simulink model "mymodel"  (R2023b)
settings: Solver=VariableStepAuto  StartTime=0.0  StopTime=10.0  RelTol=1e-3
undefined symbols (not defined in the file or in its folder): SS_lat_lo8
libraries: simulink_extras x2
settings Model: Creator=antonhendrickx  LastModifiedBy=antonhendrickx

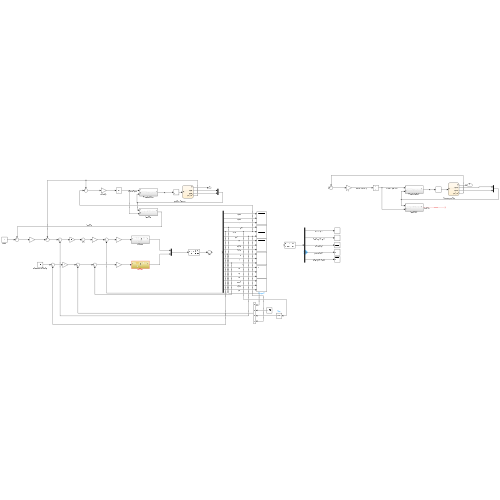
[thumbnail: Simulink's stored preview of the top-level diagram]
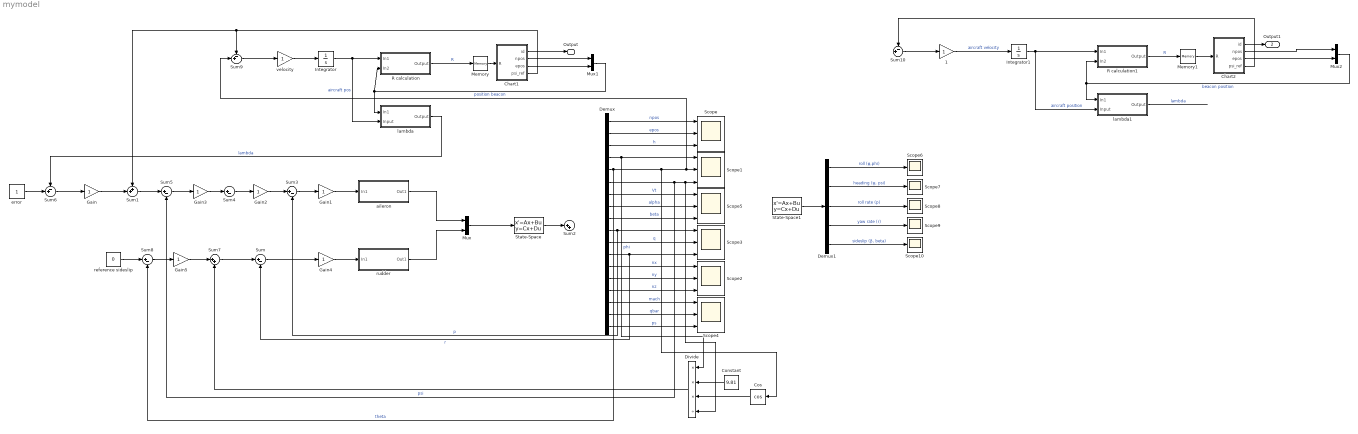
== system mymodel ==
  1 : Gain
  Chart1 : Stateflow chart  TreatAsAtomicUnit=on
  Chart2 : Stateflow chart  TreatAsAtomicUnit=on
  Constant : Constant  Value=9.81
  Cos : Trigonometry  Operator=cos
  Demux : Demux  Outputs=18
  Demux1 : Demux  Outputs=5
  Divide : Product  Inputs=***/
  Gain{,1..5} (6 alike) : Gain
  Integrator : Integrator
  Integrator1 : Integrator
  Memory : Memory
  Memory1 : Memory
  Mux : Mux  Inputs=2
  Mux1 : Mux  Inputs=2
  Mux2 : Mux  Inputs=2
  R calculation : Subsystem
  R calculation1 : Subsystem
  Scope{,1..5} (6 alike) : Scope  NumInputPorts=3
  Scope{6..10} (5 alike) : Scope
  State-Space : StateSpace  A=SS_lat_lo8.A  B=SS_lat_lo8.B  C=SS_lat_lo8.C  D=SS_lat_lo8.D  InitialCondition=0
  State-Space1 : StateSpace  InitialCondition=0
  Sum{,3..5,8} (5 alike) : Sum  Inputs=|+-
  Sum1 : Sum  Inputs=++|
  Sum10 : Sum  Inputs=-+|
  Sum2 : Sum  Inputs=|++
  Sum6 : Sum  Inputs=-+|
  Sum7 : Sum  Inputs=|++
  Sum9 : Sum  Inputs=-+|
  aileron : Subsystem
  error : Constant
  lambda : Subsystem
  lambda1 : Subsystem
  reference sideslip : Constant  Value=0
  rudder : Subsystem
  velocity : Gain
  Output : Outport
  Output1 : Outport  Port=2
  wires:
  Gain/1 -> Sum1/2
  Mux/1 -> State-Space/1
  aileron/1(Out1) -> Mux/1
  rudder/1(Out1) -> Mux/2
  Gain1/1 -> aileron/1(In1)
  Sum3/1 -> Gain1/1
  Gain2/1 -> Sum3/1
  Sum4/1 -> Gain2/1
  Gain3/1 -> Sum4/1
  Sum5/1 -> Gain3/1
  error/1 -> Sum6/2
  Sum6/1 -> Gain/1
  Sum1/1 -> Sum5/1
  Gain4/1 -> rudder/1(In1)
  Sum/1 -> Gain4/1
  Sum7/1 -> Sum/1
  Gain5/1 -> Sum7/1
  reference sideslip/1 -> Sum8/1
  Sum8/1 -> Gain5/1
  Demux/1 -> Scope/1  "npos"
  Demux/2 -> Scope/2  "epos"
  Demux/3 -> Scope/3  "h"
  Demux/4 -> Divide/1, Scope1/1  "phi"
  Demux/5 -> Sum8/2, Cos/1, Scope1/2, Sum9/2  "theta"
  Demux/6 -> Divide/4, Scope1/3, Sum5/2  "psi"
  Demux/7 -> Scope5/1  "Vt"
  Demux/8 -> Scope5/2  "alpha"
  Demux/9 -> Scope5/3  "beta"
  Demux/10 -> Sum3/2, Scope3/1  "p"
  Demux/11 -> Scope3/2  "q"
  Demux/12 -> Scope3/3, Sum/2  "r"
  Demux/13 -> Scope2/1  "nx"
  Demux/14 -> Scope2/2  "ny"
  Demux/15 -> Scope2/3  "nz"
  Demux/16 -> Scope4/1  "mach"
  Demux/17 -> Scope4/2  "qbar"
  Demux/18 -> Scope4/3  "ps"
  Chart1/1(id) -> Output/1
  Chart1/2(npos) -> Mux1/1
  Memory/1 -> Chart1/1(R)
  Chart1/3(epos) -> Mux1/2
  Sum9/1 -> velocity/1
  velocity/1 -> Integrator/1
  Integrator/1 -> lambda/2(Input), R calculation/1(In1)  "aircraft pos"
  Chart1/4(psi_ref) -> Sum9/1, Sum1/1
  Mux1/1 -> lambda/1(In1), R calculation/2(In2)  "position beacon"
  R calculation/1(Output) -> Memory/1  "R"
  lambda/1(Output) -> Sum6/1  "lambda"
  Divide/1 -> Sum7/2
  Constant/1 -> Divide/2
  Cos/1 -> Divide/3
  State-Space/1 -> Sum2/1
  Demux1/1 -> Scope6/1  "roll (φ,phi)"
  Demux1/2 -> Scope7/1  "heading (ψ, psi)"
  Demux1/3 -> Scope8/1  "roll rate (p)"
  Demux1/4 -> Scope9/1  "yaw rate (r)"
  Demux1/5 -> Scope10/1  "sideslip (β, beta)"
  State-Space1/1 -> Demux1/1
  Integrator1/1 -> lambda1/2(Input), R calculation1/1(In1)  "aircraft position"
  1/1 -> Integrator1/1  "aircraft velocity"
  Memory1/1 -> Chart2/1(R)
  R calculation1/1(Output) -> Memory1/1  "R"
  Chart2/1(id) -> Output1/1
  Chart2/2(npos) -> Mux2/1
  Chart2/3(epos) -> Mux2/2
  Chart2/4(psi_ref) -> Sum10/1
  Sum10/1 -> 1/1
  Mux2/1 -> lambda1/1(In1), R calculation1/2(In2)  "beacon position"
  lambda1/1(Output) -> ?  "lambda"

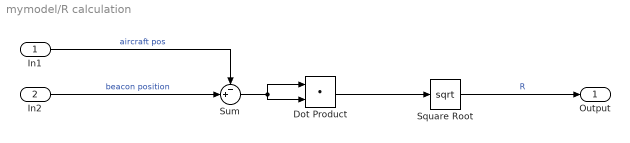
== system mymodel/R calculation ==
  In1 : Inport
  In2 : Inport  Port=2
  Dot Product : DotProduct  OutDataTypeStr=Inherit: Inherit via internal rule
  Square Root : Sqrt
  Sum : Sum  Inputs=-+|
  Output : Outport
  wires:
  In2/1 -> Sum/2  "beacon position"
  In1/1 -> Sum/1  "aircraft pos"
  Square Root/1 -> Output/1  "R"
  Dot Product/1 -> Square Root/1
  Sum/1 -> Dot Product/1, Dot Product/2

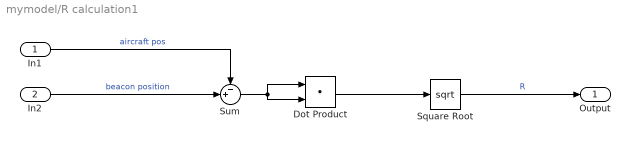
== system mymodel/R calculation1 ==
  In1 : Inport
  In2 : Inport  Port=2
  Dot Product : DotProduct  OutDataTypeStr=Inherit: Inherit via internal rule
  Square Root : Sqrt
  Sum : Sum  Inputs=-+|
  Output : Outport
  wires:
  In2/1 -> Sum/2  "beacon position"
  In1/1 -> Sum/1  "aircraft pos"
  Square Root/1 -> Output/1  "R"
  Dot Product/1 -> Square Root/1
  Sum/1 -> Dot Product/1, Dot Product/2

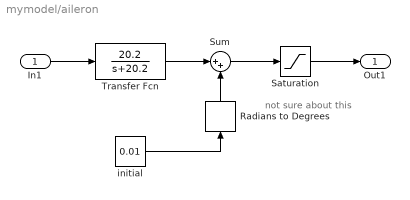
== system mymodel/aileron ==
  note: not sure about this
  In1 : Inport
  Radians to Degrees : simulink_extras/Transformations/Radians to Degrees
  Saturation : Saturate  UpperLimit=21.5  LowerLimit=-21.5
  Sum : Sum  Inputs=|++
  Transfer Fcn : TransferFcn  Numerator=[20.2]  Denominator=[1 20.2]
  initial : Constant  Value=0.01
  Out1 : Outport
  wires:
  Transfer Fcn/1 -> Sum/1
  Sum/1 -> Saturation/1
  Saturation/1 -> Out1/1
  In1/1 -> Transfer Fcn/1
  Radians to Degrees/1 -> Sum/2
  initial/1 -> Radians to Degrees/1

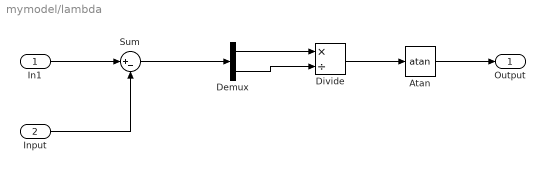
== system mymodel/lambda ==
  In1 : Inport
  Input : Inport  Port=2
  Atan : Trigonometry  Operator=atan
  Demux : Demux  Outputs=2
  Divide : Product  Inputs=*/
  Sum : Sum  Inputs=|+-
  Output : Outport
  wires:
  In1/1 -> Sum/1
  Sum/1 -> Demux/1
  Demux/2 -> Divide/2
  Demux/1 -> Divide/1
  Divide/1 -> Atan/1
  Atan/1 -> Output/1
  Input/1 -> Sum/2

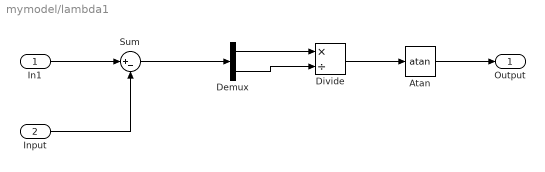
== system mymodel/lambda1 ==
  In1 : Inport
  Input : Inport  Port=2
  Atan : Trigonometry  Operator=atan
  Demux : Demux  Outputs=2
  Divide : Product  Inputs=*/
  Sum : Sum  Inputs=|+-
  Output : Outport
  wires:
  In1/1 -> Sum/1
  Sum/1 -> Demux/1
  Demux/2 -> Divide/2
  Demux/1 -> Divide/1
  Divide/1 -> Atan/1
  Atan/1 -> Output/1
  Input/1 -> Sum/2

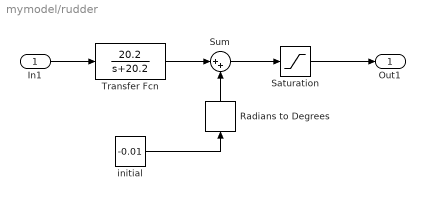
== system mymodel/rudder ==
  In1 : Inport
  Radians to Degrees : simulink_extras/Transformations/Radians to Degrees
  Saturation : Saturate  UpperLimit=30  LowerLimit=-30
  Sum : Sum  Inputs=|++
  Transfer Fcn : TransferFcn  Numerator=[20.2]  Denominator=[1 20.2]
  initial : Constant  Value=-0.01
  Out1 : Outport
  wires:
  Transfer Fcn/1 -> Sum/1
  Sum/1 -> Saturation/1
  In1/1 -> Transfer Fcn/1
  Radians to Degrees/1 -> Sum/2
  initial/1 -> Radians to Degrees/1
  Saturation/1 -> Out1/1

== stateflow chart mymodel/Chart1 ==
  settings: updateMethod=DISCRETE  sampleTime=0.1
  state beacon1
    id=1;
    npos=15000;
    epos=15000;
    psi_ref=45;
  state beacon2
    id=2;
    npos=0;
    epos=30000;
    psi_ref=135;
  state beacon3
    id=3;
    npos=-15000;
    epos=30000;
    psi_ref=180;
  state beacon4
    id=4;
    npos=-30000;
    epos=45000;
    psi_ref=135;
  state beacon5
    id=5;
    npos=0;
    epos=0;
    psi_ref=0;
  (default) -> beacon1
  beacon2 -> beacon3 : [R<5000]
  beacon3 -> beacon4 : [R<5000]
  beacon1 -> beacon2 : [R<5000]
  beacon4 -> beacon5 : [R<5000]
  beacon5 -> beacon1 : [R<5000]
  data: R input; id output; npos output; epos output; psi_ref output

== stateflow chart mymodel/Chart2 ==
  settings: updateMethod=DISCRETE  sampleTime=0.1
  state beacon1
    id=1;
    npos=15000;
    epos=15000;
    psi_ref=45;
  state beacon2
    id=2;
    npos=0;
    epos=30000;
    psi_ref=135;
  state beacon3
    id=3;
    npos=-15000;
    epos=30000;
    psi_ref=180;
  state beacon4
    id=4;
    npos=-30000;
    epos=45000;
    psi_ref=135;
  state beacon5
    id=5;
    npos=0;
    epos=0;
    psi_ref=0;
  (default) -> beacon1
  beacon2 -> beacon3 : [R<5000]
  beacon3 -> beacon4 : [R<5000]
  beacon1 -> beacon2 : [R<5000]
  beacon4 -> beacon5 : [R<5000]
  beacon5 -> beacon1 : [R<5000]
  data: R input; id output; npos output; epos output; psi_ref output
